simulink model "Mo_hinh_so_sanh_cac_phuong_phap_ham"  (R2019a)
settings: Solver=VariableStepAuto  StartTime=0.0  StopTime=10.0  RelTol=1e-3
libraries: powerlib x32
settings Model: Creator=Admin  LastModifiedBy=Admin

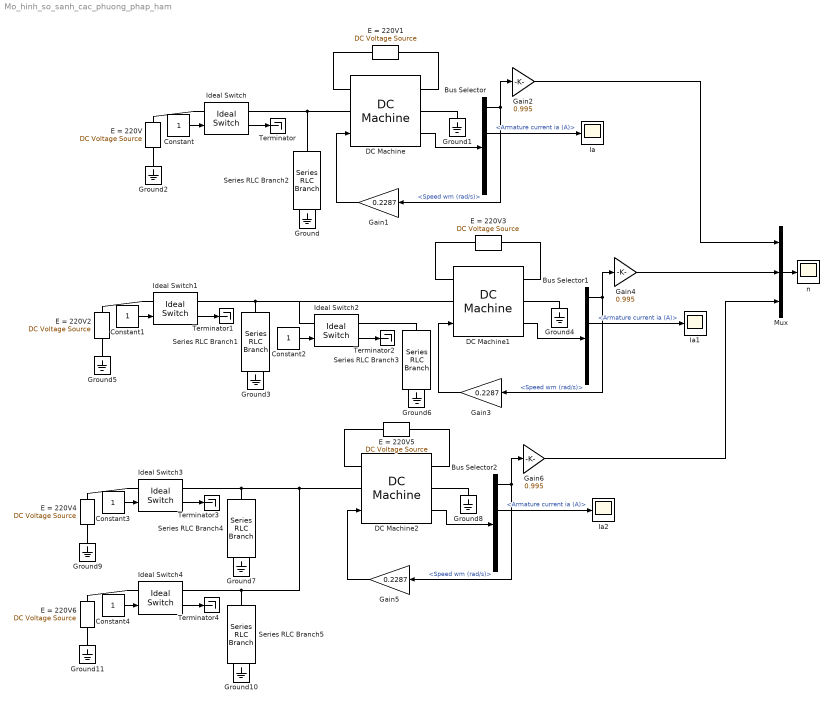
== system Mo_hinh_so_sanh_cac_phuong_phap_ham ==
  Bus Selector : BusSelector  OutputSignals=Speed wm (rad/s),Armature current ia (A),Field current if (A),Electrical torque Te (n m)
  Bus Selector1 : BusSelector  OutputSignals=Speed wm (rad/s),Armature current ia (A),Field current if (A),Electrical torque Te (n m)
  Bus Selector2 : BusSelector  OutputSignals=Speed wm (rad/s),Armature current ia (A),Field current if (A),Electrical torque Te (n m)
  Constant{,1..4} (5 alike) : Constant
  DC Machine : powerlib/Machines/DC Machine  PresetModel=No  MechanicalLoad=Torque TL  FieldType=Wound  ShowDetailedParameters=on  MeasurementBus=off  RLa=[0.2305 0.023]  RLf=[298 59.6]  Laf=1.247  MachineConstant=Torque constant (N.m/A)  Ke=1.8  Kt=1.8  J=0.28  Bm=1.58e-4  Tf=1.75  w0=1  Ifinit=1  TsPowergui=0  TsBlock=-1
  DC Machine1 : powerlib/Machines/DC Machine  PresetModel=No  MechanicalLoad=Torque TL  FieldType=Wound  ShowDetailedParameters=on  MeasurementBus=off  RLa=[0.2305 0.023]  RLf=[298 59.6]  Laf=1.247  MachineConstant=Torque constant (N.m/A)  Ke=1.8  Kt=1.8  J=0.28  Bm=1.58e-4  Tf=1.75  w0=1  Ifinit=1  TsPowergui=0  TsBlock=-1
  DC Machine2 : powerlib/Machines/DC Machine  PresetModel=No  MechanicalLoad=Torque TL  FieldType=Wound  ShowDetailedParameters=on  MeasurementBus=off  RLa=[0.2305 0.023]  RLf=[298 59.6]  Laf=1.247  MachineConstant=Torque constant (N.m/A)  Ke=1.8  Kt=1.8  J=0.28  Bm=1.58e-4  Tf=1.75  w0=1  Ifinit=1  TsPowergui=0  TsBlock=-1
  E = 220V{,1..6} (7 alike) : powerlib/Electrical Sources/DC Voltage Source  Amplitude=220  Measurements=None
  Gain1 : Gain  Gain=0.2287
  Gain2 : Gain  Gain=0.995
  Gain3 : Gain  Gain=0.2287
  Gain4 : Gain  Gain=0.995
  Gain5 : Gain  Gain=0.2287
  Gain6 : Gain  Gain=0.995
  Ground{,1..11} (12 alike) : powerlib/Elements/Ground  LConnTagsString=a
  Ia : Scope
  Ia1 : Scope
  Ia2 : Scope
  Ideal Switch{,1..4} (5 alike) : powerlib/Power Electronics/Ideal Switch  Ron=0.01  Lon=0  IC=0  Rs=inf  Cs=0  Measurements=on
  Mux : Mux  Inputs=3
  Series RLC Branch{1..2,4..5} (4 alike) : powerlib/Elements/Series RLC Branch  LConnTagsString=__new0  RConnTagsString=__new0  BranchType=R  Resistance=10000  Inductance=1e-3  SetiL0=off  InitialCurrent=0  Capacitance=1e-6  Setx0=off  InitialVoltage=0  Measurements=None
  Series RLC Branch3 : powerlib/Elements/Series RLC Branch  LConnTagsString=__new0  RConnTagsString=__new0  BranchType=R  Resistance=5  Inductance=1e-3  SetiL0=off  InitialCurrent=0  Capacitance=1e-6  Setx0=off  InitialVoltage=0  Measurements=None
  Terminator{,1..4} (5 alike) : Terminator
  "n " : Scope
  wires:
  Constant/1 -> Ideal Switch/1
  Ideal Switch/1 -> Terminator/1
  Gain1/1 -> DC Machine/1
  DC Machine/1 -> Bus Selector/1
  Bus Selector/2 -> Ia/1  "<Armature current ia (A)>"
  Bus Selector/1 -> Gain1/1, Gain2/1  "<Speed wm (rad/s)>"
  Gain3/1 -> DC Machine1/1
  Bus Selector1/1 -> Gain3/1, Gain4/1  "<Speed wm (rad/s)>"
  Bus Selector1/2 -> Ia1/1  "<Armature current ia (A)>"
  Ideal Switch1/1 -> Terminator1/1
  Constant1/1 -> Ideal Switch1/1
  DC Machine1/1 -> Bus Selector1/1
  Constant2/1 -> Ideal Switch2/1
  Ideal Switch2/1 -> Terminator2/1
  DC Machine2/1 -> Bus Selector2/1
  Constant3/1 -> Ideal Switch3/1
  Gain5/1 -> DC Machine2/1
  Bus Selector2/1 -> Gain5/1, Gain6/1  "<Speed wm (rad/s)>"
  Bus Selector2/2 -> Ia2/1  "<Armature current ia (A)>"
  Ideal Switch3/1 -> Terminator3/1
  Ideal Switch4/1 -> Terminator4/1
  Constant4/1 -> Ideal Switch4/1
  Gain2/1 -> Mux/1
  Gain4/1 -> Mux/2
  Gain6/1 -> Mux/3
  Mux/1 -> "n "/1
  connections:
  Ideal Switch/RConn1 -- Series RLC Branch2/LConn1 -- DC Machine/LConn1
  Ideal Switch/LConn1 -- E = 220V/RConn1
  Ground2/LConn1 -- E = 220V/LConn1
  E = 220V1/RConn1 -- DC Machine/LConn2
  E = 220V1/LConn1 -- DC Machine/RConn2
  DC Machine/RConn1 -- Ground1/LConn1
  Ideal Switch1/RConn1 -- Ideal Switch2/LConn1 -- DC Machine1/LConn1 -- Series RLC Branch1/LConn1
  E = 220V3/LConn1 -- DC Machine1/RConn2
  Ideal Switch1/LConn1 -- E = 220V2/RConn1
  DC Machine1/RConn1 -- Ground4/LConn1
  E = 220V3/RConn1 -- DC Machine1/LConn2
  Ground5/LConn1 -- E = 220V2/LConn1
  Ideal Switch2/RConn1 -- Series RLC Branch3/LConn1
  Ideal Switch4/RConn1 -- Series RLC Branch4/LConn1 -- Ideal Switch3/RConn1 -- DC Machine2/LConn1 -- Series RLC Branch5/LConn1
  Ground9/LConn1 -- E = 220V4/LConn1
  E = 220V5/RConn1 -- DC Machine2/LConn2
  DC Machine2/RConn1 -- Ground8/LConn1
  E = 220V5/LConn1 -- DC Machine2/RConn2
  Ideal Switch3/LConn1 -- E = 220V4/RConn1
  Ground11/LConn1 -- E = 220V6/LConn1
  Ideal Switch4/LConn1 -- E = 220V6/RConn1
